simulink library "tp120149"  (Simulink 5.1)
undefined symbols (not defined in the file): mpt_sim, nu, nx, ny, Polytope, sysStruct
settings Model: Creator=kvasnica  LastModifiedBy=michal

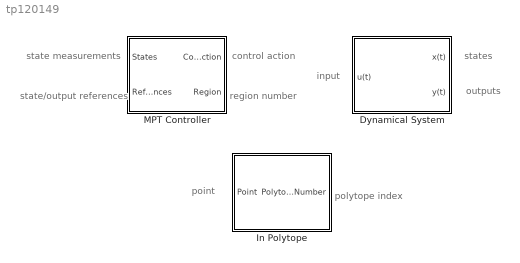
== system tp120149 ==
  note: state
      | measurements
  note: state/output
      | references
  note: control
      | action
  note: input
  note: outputs
  note: states
  note: region
      | number
  note: polytope
      | index
  note: point
  Dynamical System : Subsystem  SimViewingDevice=off  mask(Dynamical System with Constraints){sysStruct=sysStruct, x0=0, Ts=[], constr=on}
      mask prompts: sysStruct "System Structure"; x0 "Initial State"; Ts "Sampling Time (Leave empty to use default value stored in sysStruct)"; constr "Enforce Constraints"
      mask help: Gives state update and output as a function of current state and current input.
      mask init:
      | if isempty(x0)
      | 	error('Initial state must be given!');
      | end
      | if ~isfield(sysStruct,'verified')
      | 	sysStruct = mpt_verifySysStruct(sysStruct);
      | end
      | [nx,nu,ny] = mpt_sysStructInfo(sysStruct);
      | if length(x0(:))~=nx
      | 	error(['Initial state must be a ' num2str(nx) 'x1 vector!']);
      | end
      | if isfield(sysStruct, 'Ts')
      | 	ts = sysStruct.Ts;
      | else
      | 	ts = 1;
      | end
      | if isempty(Ts)
      | 	Ts = ts;
      | elseif Ts==0
      | 	Ts = ts;
      | end
      | if isempty(Ts)
      | 	error('Sampling time must be given!');
      | end
      | if Ts==0,
      | 	error('Sampling time must be greater zero!');
      | end
      settings: Permissions=ReadWrite  RTWFcnNameOpts=Auto  RTWFileNameOpts=Auto
      mask Help: This is equivalent to simulating a system using "mpt_simSys".
  In Polytope : Subsystem  AncestorBlock=mpt_sim/Polytope  SimViewingDevice=off  mask(In Polytope){P=}
      mask prompts: P "Polytope"
      mask help: Returns 0 if a given point is not inside of a given polytope, 1 otherwise.
      mask init:
      | if ~isfulldim(P),
      | 	error('Polytope must be fully dimensional!');
      | end
      | [nr, nx, abstol, H, K, nc] = mpt_getSfuncParam(P);
      settings: Permissions=ReadWrite  RTWFcnNameOpts=Auto  RTWFileNameOpts=Auto
      mask Display: image(imread('mpt_polytope.jpg'));
  MPT Controller : Subsystem  SimViewingDevice=off  mask(MPT Controller){ctrl=, Ts=[], infbreak=on}
      mask prompts: ctrl "MPT Controller Variable"; Ts "Sampling Time (Leave empty to use default value stored in controller)"; infbreak "Stop simulation if no feasible control law can be found"
      mask help: Evaluates a given explicit or on-line controller for a given state.
      mask init:
      | if isempty(ctrl)
      | 	error('No controller specified!');
      | end
      | if ~isa(ctrl, 'mptctrl')
      | 	error('Controller must be an MPTCTRL object!');
      | end
      | if cancompile(ctrl)
      |     [H, K, F, G, nc, nr, nx, nu, ny, nxt, nref, ts, dumode, tracking, abstol] = mpt_getSfuncParam(ctrl);
      |     funname = 'mpt_getInput_sfunc_parm';
      |     params = 'H, K, F, G, nc, nr, nx, nu, ny, nxt, nref, Ts, dumode, tracking, abstol, infbreak';
      | else
      |     nu = ctrl.details.dims.nu;
      | 	if isfield(ctrl.sysStruct, 'Ts'),
      | 		ts = ctrl.sysStruct.Ts;
      | 	else
      | 		ts = 1;
      | 	end
      |     funname = 'mpt_simInput_sfunc';
      |     params = 'ctrl, Ts, infbreak';
      | end
      | if isempty(Ts),
      |     Ts = ts;
      | elseif Ts==0,
      |     Ts = ts;
      | end
      | set_param(gcbh, 'MaskSelfModifiable', 'on')
      | set_param([gcb '/S-Function'], 'FunctionName', funname, 'Parameters', params);
      settings: Permissions=ReadWrite  RTWFcnNameOpts=Auto  RTWFileNameOpts=Auto
      mask Help:
      | Evaluation of an explicit control law is performed by the C-code S-function "mpt_getInput_sfunc_parm". You can also use "mpt_getInput_sfunc" function, which requires the controller to be exported to C-code using "mpt_exportc".
      | 
      | Evaluation of an on-line controller is performed by calling mpt_getInpit.m
      mask Display: image(imread('mpt_ctrl.jpg'));

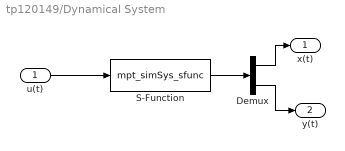
== system tp120149/Dynamical System ==
  u(t) : Inport  Port=1  PortDimensions=-1  SampleTime=-1  DataType=auto
      settings: SignalType=auto
  Demux : Demux  Outputs=[nx ny]  BusSelectionMode=off
  S-Function : S-Function  FunctionName=mpt_simSys_sfunc  Parameters=sysStruct,x0,Ts,nx,nu,ny,constr  PortCounts=[]  SFunctionModules=''
  x(t) : Outport  Port=1
  y(t) : Outport  Port=2
  wires:
  u(t)/1 -> S-Function/1
  S-Function/1 -> Demux/1
  Demux/1 -> x(t)/1
  Demux/2 -> y(t)/1

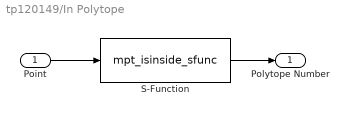
== system tp120149/In Polytope ==
  Point : Inport  Port=1  PortDimensions=-1  SampleTime=-1  DataType=auto
      settings: SignalType=auto
  S-Function : S-Function  FunctionName=mpt_isinside_sfunc  Parameters=nr, nx, abstol, H, K, nc  PortCounts=[]  SFunctionModules=''
  Polytope Number : Outport  Port=1
  wires:
  S-Function/1 -> Polytope Number/1
  Point/1 -> S-Function/1

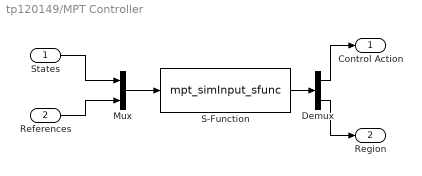
== system tp120149/MPT Controller ==
  States : Inport  Port=1  PortDimensions=-1  SampleTime=-1  DataType=auto
      settings: SignalType=auto
  References : Inport  Port=2  PortDimensions=-1  SampleTime=-1  DataType=auto
      settings: SignalType=auto
  Demux : Demux  Outputs=[nu 1]  BusSelectionMode=off
  Mux : Mux  Inputs=2
  S-Function : S-Function  FunctionName=mpt_simInput_sfunc  Parameters=ctrl, Ts  PortCounts=[]  SFunctionModules=''
  Control Action : Outport  Port=1
  Region : Outport  Port=2
  wires:
  Mux/1 -> S-Function/1
  States/1 -> Mux/1
  References/1 -> Mux/2
  S-Function/1 -> Demux/1
  Demux/1 -> Control Action/1
  Demux/2 -> Region/1
